simulink model "Pwer_electronics_partC"  (R2024b)
settings: Solver=VariableStepAuto  StartTime=0.0  StopTime=0.04  RelTol=1e-3
libraries: spsMeanLib x3, spsDiodeLib x2, spsRMSLib x2, spsVoltageMeasurementLib x2, spsACVoltageSourceLib x1, spsCurrentMeasurementLib x1, spsFourierLib x1, spsSeriesRLCBranchLib x1, sps_lib x1
settings Model: Creator=MTMTAD006  LastModifiedBy=MTMTAD006

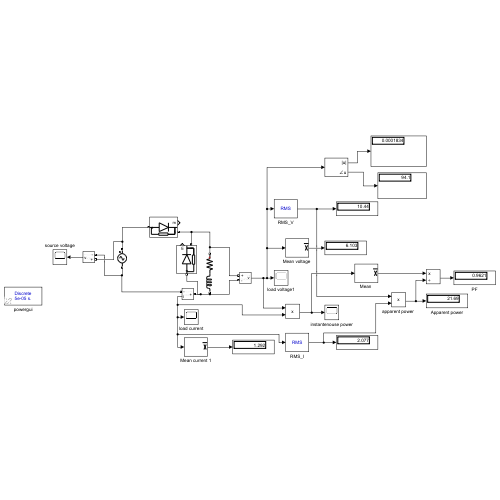
[thumbnail: Simulink's stored preview of the top-level diagram]
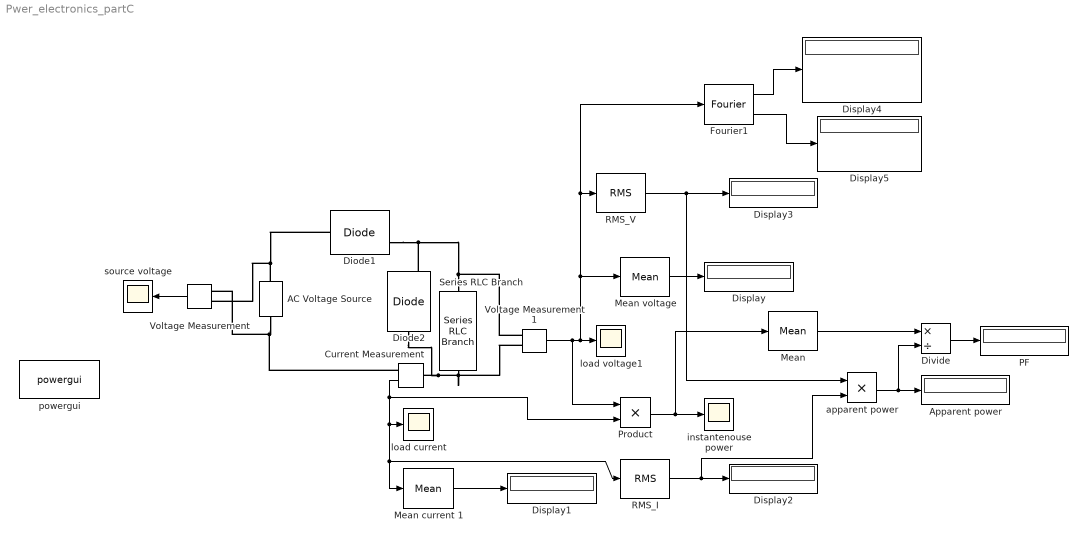
== system Pwer_electronics_partC ==
  AC Voltage Source : spsACVoltageSourceLib/AC Voltage Source  Amplitude=15*sqrt(2)  Phase=0  Frequency=50  SampleTime=0  Measurements=None  BusType=swing  Pref=10e3  Qref=0  Qmin=-inf  Qmax=+inf
  Apparent power : Display
  Current Measurement : spsCurrentMeasurementLib/Current Measurement  PhasorSimulation=off  OutputType=Complex  PSBequivalent=0
  Diode1 : spsDiodeLib/Diode  Ron=0.001  Lon=0  Vf=0  IC=0  UseSnubber=0  Rs=5000  Cs=250e-9  Measurements=on
  Diode2 : spsDiodeLib/Diode  Ron=0.001  Lon=0  Vf=0  IC=0  UseSnubber=0  Rs=5000  Cs=250e-9  Measurements=on
  Display{,1..5} (6 alike) : Display
  Divide : Product  Inputs=*/
  Fourier1 : spsFourierLib/Fourier  Freq=50  n=5  InInit=[0, 0]  Ts=0
  "Mean " : spsMeanLib/Mean  Freq=60  Vinit=0  Ts=0
  Mean current 1 : spsMeanLib/Mean  Freq=60  Vinit=0  Ts=0
  "Mean voltage " : spsMeanLib/Mean  Freq=60  Vinit=0  Ts=0
  PF : Display
  Product : Product
  RMS_I : spsRMSLib/RMS  TrueRMS=on  Freq=60  RMSInit=120  Ts=0
  RMS_V : spsRMSLib/RMS  TrueRMS=on  Freq=60  RMSInit=120  Ts=0
  Series RLC Branch : spsSeriesRLCBranchLib/Series RLC Branch  LConnTagsString=__new0  RConnTagsString=__new0  BranchType=RL  Resistance=5  Inductance=7e-3  SetiL0=off  InitialCurrent=0  Capacitance=1e-6  Setx0=off  InitialVoltage=0  Measurements=None
  Voltage Measurement : spsVoltageMeasurementLib/Voltage Measurement  PhasorSimulation=off  OutputType=Complex  PSBequivalent=0
  Voltage Measurement1 : spsVoltageMeasurementLib/Voltage Measurement  PhasorSimulation=off  OutputType=Complex  PSBequivalent=0
  "apparent power " : Product
  instantenouse power : Scope
  load current : Scope
  load voltage1 : Scope
  powergui : sps_lib/powergui  Priority=1  SimulationMode=Discrete  SampleTime=50e-6  frequency=60  Iterations=50  frequencyindice=50  Pbase=100e6  ErrMax=1e-4  UnitsV=kV  UnitsW=MW  buscounter=0  FunctionMessages=off  echomessages=off  EnableUseOfTLC=off  CurrentSourceSwitches=off  DisableSnubberDevices=off  DisableRonSwitches=off  DisableVfSwitches=off  DisplayEquations=off  AutomaticDiscreteSolvers=off  SolverType=Tustin/Backward Euler (TBE)  Interpol=off  ExternalGateDelay=off  methode=off  Ts=100  x0status=blocks  SPID=on  SwTol=0  HookPort=off  NonlinearTolerance=1e-4  nMaxIteration=100  ContinueOnMaxIteration=off  RestoreLinks=warning  ResistiveCurrentMeasurement=off  Frange=[0:2:500]  Ylog=off  Xlog=on  ShowGrid=off  save=off  variable=ZData  structure=0  ZoomFFT=off  StartTime=0.0  cycles=1  DisplayStyle=1  fundamental=60  FreqAxis=off  MaxFrequency=1000  frequencyindicesteady=1  RmsSteady=1  display=off
  source voltage : Scope
  wires:
  Voltage Measurement/1 -> source voltage/1
  Voltage Measurement1/1 -> Product/1, Fourier1/1, RMS_V/1, "Mean voltage "/1, load voltage1/1
  Current Measurement/1 -> Product/2, RMS_I/1, Mean current 1/1, load current/1
  Product/1 -> "Mean "/1, instantenouse power/1
  "Mean voltage "/1 -> Display/1
  Mean current 1/1 -> Display1/1
  RMS_I/1 -> "apparent power "/2, Display2/1
  RMS_V/1 -> Display3/1, "apparent power "/1
  "apparent power "/1 -> Divide/2, Apparent power/1
  Divide/1 -> PF/1
  "Mean "/1 -> Divide/1
  Fourier1/1 -> Display4/1
  Fourier1/2 -> Display5/1
  connections:
  AC Voltage Source/RConn1 -- Diode1/LConn1 -- Voltage Measurement/LConn1
  Series RLC Branch/LConn1 -- Diode2/RConn1 -- Diode1/RConn1 -- Voltage Measurement1/LConn1
  AC Voltage Source/LConn1 -- Current Measurement/RConn1 -- Voltage Measurement/LConn2
  Voltage Measurement1/LConn2 -- Series RLC Branch/RConn1 -- Diode2/LConn1 -- Current Measurement/LConn1
